simulink model "uz_codegen"  (R2021a)
settings: Solver=FixedStepDiscrete  StartTime=0.0  StopTime=50  RelTol=1e-3  EnableMultiTasking=on
PreLoadFcn:
  | uz_setCodegenPaths
model workspace (MATLAB code in the model file):
  | cmdLim = Simulink.Parameter;
  | cmdLim.Value = 15;
  | cmdLim.Description = 'Limit for controlling the maximum surface command angle.';
  | cmdLim.Min = 0;
  | cmdLim.Max = 90;
  | cmdLim.DocUnits = 'deg';
  | 
  | dispGain = Simulink.Parameter;
  | dispGain.Value = 0.75;
  | dispGain.Description = 'Gain applied to the displacement error.';
  | dispGain.Min = 0;
  | dispGain.Max = [];
  | dispGain.DocUnits = 'deg/sec/deg';
  | 
  | dispLim = Simulink.Parameter;
  | dispLim.Value = 30;
  | dispLim.Description = 'Limit for controlling the maximum commanded angle.';
  | dispLim.Min = 0;
  | dispLim.Max = 180;
  | dispLim.DocUnits = 'deg';
  | 
  | intGain = Simulink.Parameter;
  | intGain.Value = 0.5;
  | intGain.Description = 'Gain applied to the integral error.';
  | intGain.Min = 0;
  | intGain.Max = [];
  | intGain.DocUnits = 'deg/sec/deg/sec';
  | 
  | intLim = Simulink.Parameter;
  | intLim.Value = 5;
  | intLim.Description = 'Limit for controlling the maximum commanded angle.';
  | intLim.Min = 0;
  | intLim.Max = 90;
  | intLim.DocUnits = 'deg';
  | 
  | rateGain = Simulink.Parameter;
  | rateGain.Value = 2;
  | rateGain.Description = 'Gain applied to the rate error.';
  | rateGain.Min = 0;
  | rateGain.Max = [];
  | rateGain.DocUnits = 'deg/deg/sec';
  | 
  | rateLim = Simulink.Parameter;
  | rateLim.Value = 6;
  | rateLim.Description = 'Limit for controlling the maximum commanded angle.';
  | rateLim.Min = 0;
  | rateLim.Max = 180;
  | rateLim.DocUnits = 'deg/sec';
  | 
  | hdgGain = Simulink.Parameter;
  | hdgGain.Value = 0.015;
values from neighbouring files (symbols this model uses):
  I_max = 100    [PMSM_01_Parameter.m]
  Iq_Intersection_Wb = sqrt(I_max^2 - Id_Intersection_Wb^2)    [Plot_MMPA.m]
  Ki_IdController = R/Ld    (= 3749.81250937)    [PMSM_01_Parameter.m]
  Ki_IqController = R/Lq    (= 2500)    [PMSM_01_Parameter.m]
  Ki_SpeedController = Kp_IqController/(Lq*damping_factor^2)    (= 174.532925199)    [PMSM_01_Parameter.m]
  Ki_TorqueController = 1/(4*T_summe_Torque)    (= 714.285714286)    [PMSM_01_Parameter.m]
  Kp_IdController = Ld*2*pi*BW    (= 0.0670239943087)    [PMSM_01_Parameter.m]
  Kp_IqController = Lq*2*pi*BW    (= 0.100530964915)    [PMSM_01_Parameter.m]
  Kp_SpeedController = Kp_IqController/(Lq*damping_factor*K)    (= 2.90111828368)    [PMSM_01_Parameter.m]
  Kp_TorqueController = T1_Torque/(2*T_summe_Torque)    (= 0.373999125427)    [PMSM_01_Parameter.m]
  Ld = 0.6667*Lq    (= 1.06672e-05)    [PMSM_01_Parameter.m]
  List_Iq_Intersection_Speed = zeros(length(List_wEl_Intersection_Speed),1)    [Plot_MMPA.m]
  List_Iq_Torque = zeros(length(List_M_const),1)    [Plot_MMPA.m]
  List_Iq_Torque_Imax = List_Iq_Torque_Imax(List_Iq_Torque_Imax ~= -1)    [Plot_MMPA.m]
  List_M_const = 0:0.5:10    [Plot_MMPA.m]
  List_M_Imax = List_M_const(List_Iq_Torque_Imax ~= -1)    [Plot_MMPA.m]
  List_wEl_Intersection_Speed = linspace(n_cut,n_max,15)    [Plot_MMPA.m]
  Lq = 16e-6    (= 1.6e-05)    [PMSM_01_Parameter.m]
  n_cut = w_b*30/(pi*zp)    [Plot_MMPA.m]
  psi_pm = 0.0030    (= 0.003)    [PMSM_01_Parameter.m]
  R = 0.040    (= 0.04)    [PMSM_01_Parameter.m]
  T_controller = 1/f_CurrentController    (= 0.0001)    [PMSM_01_Parameter.m]
  T_speedController = T_controller    (= 0.0001)    [PMSM_01_Parameter.m]
  U_DC = 46    [PMSM_01_Parameter.m]
  U_maxDQ = U_DC/sqrt(3)    [PMSM_01_Parameter.m]
  zp = 21    [PMSM_01_Parameter.m]
undefined symbols (not defined in the file or in its folder): denum_Gd_speed, denum_Gd_trq, num_Gd_speed, num_Gd_trq
libraries: pid_lib x8, simulink x7, spsabctodq0Lib x2, spsdq0toAlphaBetaZeroLib x2
(part 2 of 2)

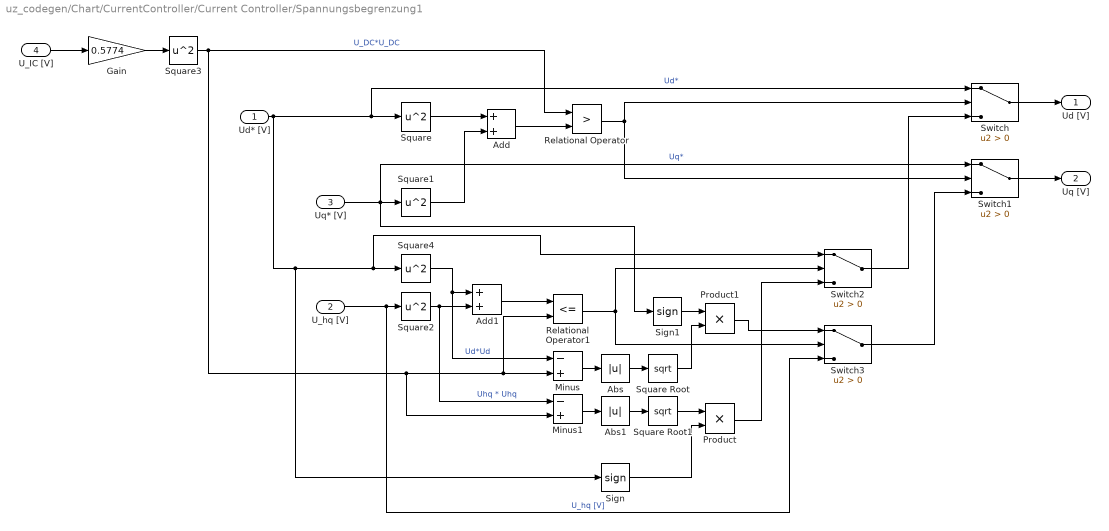
== system uz_codegen/Chart/CurrentController/Current Controller/Spannungsbegrenzung1 ==
  Ud* [V] : Inport
  U_hq [V] : Inport  Port=2
  Uq* [V] : Inport  Port=3
  U_IC [V] : Inport  Port=4
  Abs : Abs
  Abs1 : Abs
  Add : Sum
  Add1 : Sum
  Gain : Gain  Gain=0.5774
  Minus : Sum  Inputs=-+
  Minus1 : Sum  Inputs=-+
  Product : Product
  Product1 : Product
  Relational Operator : RelationalOperator  Operator=>  OutDataTypeStr=boolean  RndMeth=Simplest
  Relational Operator1 : RelationalOperator  Operator=<=  OutDataTypeStr=boolean  RndMeth=Simplest
  Sign : Signum
  Sign1 : Signum
  Square{,1..4} (5 alike) : Math  Operator=square  SaturateOnIntegerOverflow=on
  Square Root : Sqrt  SaturateOnIntegerOverflow=on
  Square Root1 : Sqrt  SaturateOnIntegerOverflow=on
  Switch{,1..3} (4 alike) : Switch  Criteria=u2 > Threshold
  Ud [V] : Outport
  Uq [V] : Outport  Port=2
  wires:
  Ud* [V]/1 -> Sign/1, Switch2/1, Square4/1, Switch/1, Square/1  "Ud*"
  Uq* [V]/1 -> Switch1/1, Sign1/1, Square1/1  "Uq*"
  U_hq [V]/1 -> Switch3/3, Square2/1  "U_hq [V]"
  U_IC [V]/1 -> Gain/1
  Square1/1 -> Add/2
  Square/1 -> Add/1
  Square3/1 -> Minus1/2, Minus/2, Relational Operator1/2, Relational Operator/1  "U_DC*U_DC"
  Add/1 -> Relational Operator/2
  Switch/1 -> Ud [V]/1
  Relational Operator/1 -> Switch1/2, Switch/2
  Switch1/1 -> Uq [V]/1
  Square2/1 -> Minus1/1, Add1/2  "Uhq * Uhq"
  Square4/1 -> Minus/1, Add1/1  "Ud*Ud"
  Add1/1 -> Relational Operator1/1
  Relational Operator1/1 -> Switch2/2, Switch3/2
  Switch2/1 -> Switch/3
  Switch3/1 -> Switch1/3
  Minus/1 -> Abs/1
  Square Root/1 -> Product1/2
  Minus1/1 -> Abs1/1
  Square Root1/1 -> Product/1
  Abs1/1 -> Square Root1/1
  Abs/1 -> Square Root/1
  Gain/1 -> Square3/1
  Sign/1 -> Product/2
  Product/1 -> Switch2/3
  Sign1/1 -> Product1/1
  Product1/1 -> Switch3/1

== system uz_codegen/Chart/SpeedController/speed controller/MMPA_Controller ==
  flg_speedControl : Inport
  n_soll : Inport  Port=2
  n_ist : Inport  Port=3
  id_ref : Inport  Port=4
  iq_ref : Inport  Port=5
  Discrete Transfer Fcn : DiscreteTransferFcn  Numerator=num_Gd_trq  Denominator=denum_Gd_trq
  PID Controller : pid_lib/PID Controller  Controller=PI  Form=Ideal  TimeDomain=Discrete-time  UseExternalTs=off  SampleTime=-1  IntegratorMethod=Forward Euler  FilterMethod=Forward Euler  ControllerParametersSource=internal  P=Kp_TorqueController  I=Ki_TorqueController  D=0  UseFilter=on  N=100  TunerSelectOption=Transfer Function Based (PID Tuner App)  InitialConditionSource=internal  InitialConditionForIntegrator=0  InitialConditionForFilter=0  DifferentiatorICPrevScaledInput=0  ExternalReset=none  TrackingMode=off  Kt=1  LimitOutput=on  SatLimitsSource=internal  UpperSaturationLimit=8  LowerSaturationLimit=-8  LinearizeAsGain=on  AntiWindupMode=clamping  Kb=1  POutMin=[]  POutMax=[]  IOutMin=[]  IOutMax=[]  DOutMin=[]  DOutMax=[]  NOutMin=[]  NOutMax=[]  SumOutMin=[]  SumOutMax=[]  SaturationOutMin=[]  SaturationOutMax=[]  PParamMin=[]  PParamMax=[]  IParamMin=[]  IParamMax=[]  DParamMin=[]  DParamMax=[]  NParamMin=[]  NParamMax=[]  KbParamMin=[]  KbParamMax=[]  KtParamMin=[]  KtParamMax=[]  KbOutMin=[]  KbOutMax=[]  KtOutMin=[]  KtOutMax=[]  IntegratorOutMin=[]  IntegratorOutMax=[]  FilterOutMin=[]  FilterOutMax=[]  SumI1OutMin=[]  SumI1OutMax=[]  SumI2OutMin=[]  SumI2OutMax=[]  SumI3OutMin=[]  SumI3OutMax=[]  SumI4OutMin=[]  SumI4OutMax=[]  SumDOutMin=[]  SumDOutMax=[]  DifferentiatorOutMin=[]  DifferentiatorOutMax=[]  FilterDiffOutCoefMin=[]  FilterDiffOutCoefMax=[]  ReciprocalOutMin=[]  ReciprocalOutMax=[]  SumDenOutMin=[]  SumDenOutMax=[]  SumNumOutMin=[]  SumNumOutMax=[]  DivideOutMin=[]  DivideOutMax=[]  UdiffTsProdOutMin=[]  UdiffTsProdOutMax=[]  NTsProdOutMin=[]  NTsProdOutMax=[]  UintegralTsProdOutMin=[]  UintegralTsProdOutMax=[]  UngainTsProdOutMin=[]  UngainTsProdOutMax=[]  IntegratorContinuousStateAttributes=''  IntegratorStateMustResolveToSignalObject=off  IntegratorRTWStateStorageClass=Auto  FilterContinuousStateAttributes=''  FilterStateMustResolveToSignalObject=off  FilterRTWStateStorageClass=Auto  ParallelPVariant=Passthrough  IdealPVariant=InternalParameters  IVariant=InternalParameters  DVariant=Disabled  IntegratorVariant=Discrete  SatVariant=Enabled  AWVariant=DiscClampingIdeal  PCopyVariant=InternalParamsIdeal  TRVariant=Disabled  FdbkBlocksVariant=Forward  IdealPFdbkVariant=Disabled  SatFdbkVariant=Disabled  DerivativeFilterVariant=Disabled  NVariant=Disabled  NCopyVariant=Disabled_SignalSpec  FilterICVariant=Disabled  IntegratorICVariant=InternalICs  ExternalResetVariant=Disabled  TRSumVariant=Passthrough  SumFdbkVariant=Disabled  SumVariant=Sum_PI  TsampFilterVariant=InternalTs  TsampNgainVariant=Passthrough  TsampIntegralVariant=Passthrough  ExternalSaturationOutDataTypeStr=Inherit: Same as second input
  Scope : Scope  NumInputPorts=2
  Scope1 : Scope
  Subsystem : Subsystem
  Sum : Sum  Inputs=|+-
  Switch : Switch  Criteria=u2 > Threshold
  Switch1 : Switch  Criteria=u2 > Threshold
  id_soll : Outport
  Iq_soll : Outport  Port=2
  wires:
  Subsystem/1(Iq) -> Scope/1, Switch1/1
  PID Controller/1 -> Scope1/1, Subsystem/1(M_soll)  "M_soll"
  n_soll/1 -> Discrete Transfer Fcn/1
  flg_speedControl/1 -> Switch/2, Switch1/2
  n_ist/1 -> Sum/2, Subsystem/2(n_ist)
  iq_ref/1 -> Switch1/3
  id_ref/1 -> Switch/3
  Sum/1 -> PID Controller/1
  Subsystem/2(Id) -> Scope/2, Switch/1
  Discrete Transfer Fcn/1 -> Sum/1
  Switch1/1 -> Iq_soll/1
  Switch/1 -> id_soll/1

== system uz_codegen/Chart/SpeedController/speed controller/Subsystem ==
  flg_fieldWeakening : Inport
  id_ref : Inport  Port=2
  n_soll : Inport  Port=3
  flg_speedControl : Inport  Port=4
  n_ist : Inport  Port=5
  iq_ref : Inport  Port=6
  Constant : Constant  Value=0
  PID Controller : pid_lib/PID Controller  Controller=PI  Form=Ideal  TimeDomain=Discrete-time  UseExternalTs=off  SampleTime=-1  IntegratorMethod=Forward Euler  FilterMethod=Forward Euler  ControllerParametersSource=internal  P=Kp_SpeedController  I=Ki_SpeedController  D=0  UseFilter=on  N=100  TunerSelectOption=Transfer Function Based (PID Tuner App)  InitialConditionSource=internal  InitialConditionForIntegrator=0  InitialConditionForFilter=0  DifferentiatorICPrevScaledInput=0  ExternalReset=none  TrackingMode=off  Kt=1  LimitOutput=on  SatLimitsSource=internal  UpperSaturationLimit=I_max  LowerSaturationLimit=-I_max  LinearizeAsGain=on  AntiWindupMode=clamping  Kb=1  POutMin=[]  POutMax=[]  IOutMin=[]  IOutMax=[]  DOutMin=[]  DOutMax=[]  NOutMin=[]  NOutMax=[]  SumOutMin=[]  SumOutMax=[]  SaturationOutMin=[]  SaturationOutMax=[]  PParamMin=[]  PParamMax=[]  IParamMin=[]  IParamMax=[]  DParamMin=[]  DParamMax=[]  NParamMin=[]  NParamMax=[]  KbParamMin=[]  KbParamMax=[]  KtParamMin=[]  KtParamMax=[]  KbOutMin=[]  KbOutMax=[]  KtOutMin=[]  KtOutMax=[]  IntegratorOutMin=[]  IntegratorOutMax=[]  FilterOutMin=[]  FilterOutMax=[]  SumI1OutMin=[]  SumI1OutMax=[]  SumI2OutMin=[]  SumI2OutMax=[]  SumI3OutMin=[]  SumI3OutMax=[]  SumI4OutMin=[]  SumI4OutMax=[]  SumDOutMin=[]  SumDOutMax=[]  DifferentiatorOutMin=[]  DifferentiatorOutMax=[]  FilterDiffOutCoefMin=[]  FilterDiffOutCoefMax=[]  ReciprocalOutMin=[]  ReciprocalOutMax=[]  SumDenOutMin=[]  SumDenOutMax=[]  SumNumOutMin=[]  SumNumOutMax=[]  DivideOutMin=[]  DivideOutMax=[]  UdiffTsProdOutMin=[]  UdiffTsProdOutMax=[]  NTsProdOutMin=[]  NTsProdOutMax=[]  UintegralTsProdOutMin=[]  UintegralTsProdOutMax=[]  UngainTsProdOutMin=[]  UngainTsProdOutMax=[]  IntegratorContinuousStateAttributes=''  IntegratorStateMustResolveToSignalObject=off  IntegratorRTWStateStorageClass=Auto  FilterContinuousStateAttributes=''  FilterStateMustResolveToSignalObject=off  FilterRTWStateStorageClass=Auto  ParallelPVariant=Passthrough  IdealPVariant=InternalParameters  IVariant=InternalParameters  DVariant=Disabled  IntegratorVariant=Discrete  SatVariant=Enabled  AWVariant=DiscClampingIdeal  PCopyVariant=InternalParamsIdeal  TRVariant=Disabled  FdbkBlocksVariant=Forward  IdealPFdbkVariant=Disabled  SatFdbkVariant=Disabled  DerivativeFilterVariant=Disabled  NVariant=Disabled  NCopyVariant=Disabled_SignalSpec  FilterICVariant=Disabled  IntegratorICVariant=InternalICs  ExternalResetVariant=Disabled  TRSumVariant=Passthrough  SumFdbkVariant=Disabled  SumVariant=Sum_PI  TsampFilterVariant=InternalTs  TsampNgainVariant=Passthrough  TsampIntegralVariant=Passthrough  ExternalSaturationOutDataTypeStr=Inherit: Same as second input
  Sum : Sum  Inputs=|+-
  Switch : Switch  Criteria=u2 > Threshold
  Switch1 : Switch  Criteria=u2 > Threshold
  id_soll : Outport
  iq_soll : Outport  Port=2
  wires:
  iq_ref/1 -> Switch1/3
  n_ist/1 -> Sum/2
  id_ref/1 -> Switch/3
  flg_fieldWeakening/1 -> Switch/2
  PID Controller/1 -> Switch1/1
  Sum/1 -> PID Controller/1
  flg_speedControl/1 -> Switch1/2
  n_soll/1 -> Sum/1
  Switch/1 -> id_soll/1
  Switch1/1 -> iq_soll/1
  Constant/1 -> Switch/1

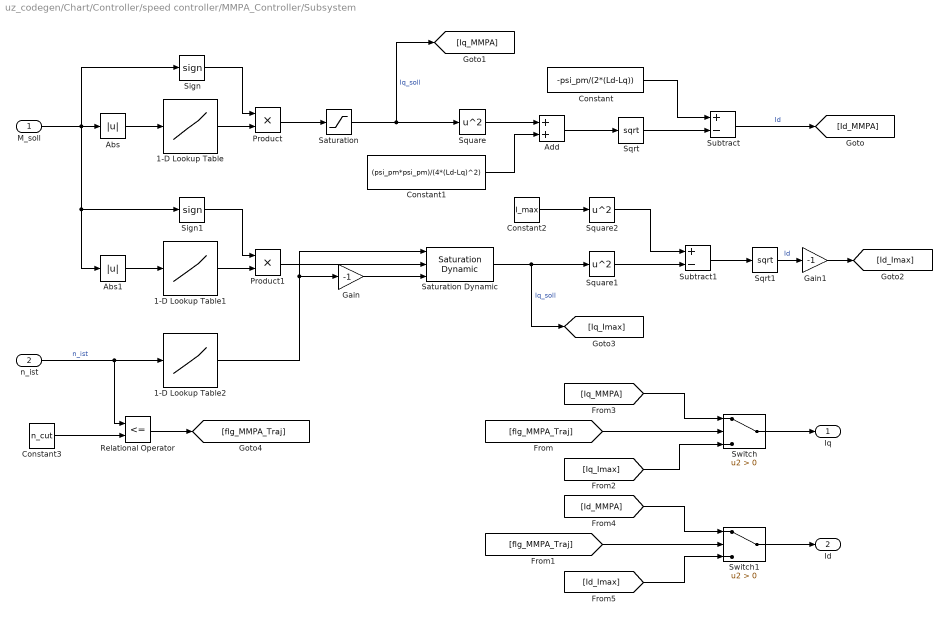
== system uz_codegen/Chart/Controller/speed controller/MMPA_Controller/Subsystem ==
  M_soll : Inport
  n_ist : Inport  Port=2
  1-D Lookup Table : Lookup_n-D  NumberOfTableDimensions=1  BreakpointsForDimension1=List_M_const  Table=List_Iq_Torque  InternalRulePriority=Speed  RndMeth=Simplest  InputSameDT=on
  1-D Lookup Table1 : Lookup_n-D  NumberOfTableDimensions=1  BreakpointsForDimension1=List_M_Imax  Table=List_Iq_Torque_Imax  InternalRulePriority=Speed  RndMeth=Simplest  InputSameDT=on
  1-D Lookup Table2 : Lookup_n-D  NumberOfTableDimensions=1  BreakpointsForDimension1=List_wEl_Intersection_Speed  Table=List_Iq_Intersection_Speed  InternalRulePriority=Speed  RndMeth=Simplest  InputSameDT=on
  Abs : Abs
  Abs1 : Abs
  Add : Sum
  Constant : Constant  Value=-psi_pm/(2*(Ld-Lq))
  Constant1 : Constant  Value=(psi_pm*psi_pm)/(4*(Ld-Lq)^2)
  Constant2 : Constant  Value=I_max
  Constant3 : Constant  Value=n_cut
  Gain : Gain  Gain=-1
  Gain1 : Gain  Gain=-1
  Product : Product
  Product1 : Product
  Relational Operator : RelationalOperator  Operator=<=  OutDataTypeStr=boolean  RndMeth=Simplest
  Saturation : Saturate  UpperLimit=Iq_Intersection_Wb  LowerLimit=-Iq_Intersection_Wb
  Saturation Dynamic : simulink/Discontinuities/Saturation Dynamic  OutMin=[]  OutMax=[]  OutDataTypeStr=Inherit: Same as second input  OutDataType=fixdt(1, 16)  OutScaling=2^-10  DoSatur=off
  Sign : Signum
  Sign1 : Signum
  Sqrt : Sqrt  SaturateOnIntegerOverflow=on
  Sqrt1 : Sqrt  SaturateOnIntegerOverflow=on
  Square : Math  Operator=square  SaturateOnIntegerOverflow=on
  Square1 : Math  Operator=square  SaturateOnIntegerOverflow=on
  Square2 : Math  Operator=square  SaturateOnIntegerOverflow=on
  Subtract : Sum  Inputs=+-
  Subtract1 : Sum  Inputs=+-
  Switch : Switch  Criteria=u2 > Threshold
  Switch1 : Switch  Criteria=u2 > Threshold
  Iq : Outport
  Id : Outport  Port=2
  wires:
  1-D Lookup Table/1 -> Product/2
  Abs/1 -> 1-D Lookup Table/1
  Product/1 -> Saturation/1
  Sign/1 -> Product/1
  Saturation/1 -> [Iq_MMPA], Square/1  "Iq_soll"
  Square/1 -> Add/1
  Constant1/1 -> Add/2
  Add/1 -> Sqrt/1
  Sqrt/1 -> Subtract/2
  Constant/1 -> Subtract/1
  Subtract/1 -> [Id_MMPA]  "Id"
  Abs1/1 -> 1-D Lookup Table1/1
  Sign1/1 -> Product1/1
  Product1/1 -> Saturation Dynamic/2
  M_soll/1 -> Abs/1, Sign1/1, Abs1/1, Sign/1
  1-D Lookup Table1/1 -> Product1/2
  n_ist/1 -> Relational Operator/1, 1-D Lookup Table2/1  "n_ist"
  1-D Lookup Table2/1 -> Gain/1, Saturation Dynamic/1
  Gain/1 -> Saturation Dynamic/3
  Saturation Dynamic/1 -> [Iq_Imax], Square1/1  "Iq_soll"
  Constant2/1 -> Square2/1
  Square1/1 -> Subtract1/2
  Square2/1 -> Subtract1/1
  Subtract1/1 -> Sqrt1/1
  Sqrt1/1 -> Gain1/1  "Id"
  Constant3/1 -> Relational Operator/2
  Relational Operator/1 -> [flg_MMPA_Traj]
  [flg_MMPA_Traj] -> Switch/2
  [flg_MMPA_Traj] -> Switch1/2
  [Iq_Imax] -> Switch/3
  [Iq_MMPA] -> Switch/1
  [Id_MMPA] -> Switch1/1
  [Id_Imax] -> Switch1/3
  Switch1/1 -> Id/1
  Switch/1 -> Iq/1
  Gain1/1 -> [Id_Imax]

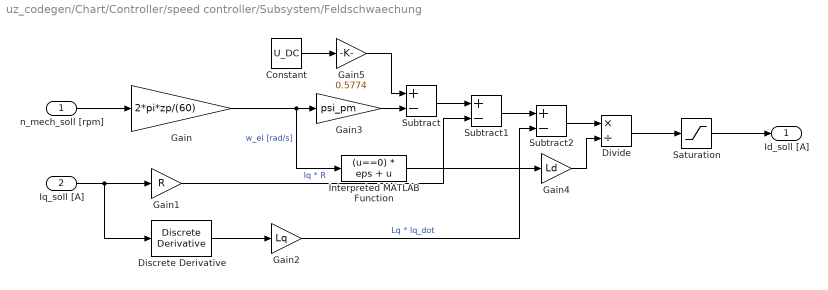
== system uz_codegen/Chart/Controller/speed controller/Subsystem/Feldschwaechung ==
  n_mech_soll [rpm] : Inport
  Iq_soll [A] : Inport  Port=2
  Constant : Constant  Value=U_DC
  Discrete Derivative : simulink/Discrete/Discrete Derivative  gainval=1.0  ICPrevScaledInput=0.0  OutMin=[]  OutMax=[]  OutDataType=fixdt(1, 16)  OutScaling=2^-10  DoSatur=off
  Divide : Product  Inputs=*/
  Gain : Gain  Gain=2*pi*zp/(60)
  Gain1 : Gain  Gain=R
  Gain2 : Gain  Gain=Lq
  Gain3 : Gain  Gain=psi_pm
  Gain4 : Gain  Gain=Ld
  Gain5 : Gain  Gain=0.5774
  Interpreted MATLAB Function : MATLABFcn  MATLABFcn=(u==0) * eps + u
  Saturation : Saturate  UpperLimit=0  LowerLimit=-I_max
  Subtract : Sum  Inputs=+-
  Subtract1 : Sum  Inputs=+-
  Subtract2 : Sum  Inputs=+-
  Id_soll [A] : Outport
  wires:
  n_mech_soll [rpm]/1 -> Gain/1
  Gain/1 -> Interpreted MATLAB Function/1, Gain3/1  "w_el [rad/s]"
  Gain1/1 -> Subtract1/2  "Iq * R"
  Iq_soll [A]/1 -> Discrete Derivative/1, Gain1/1
  Discrete Derivative/1 -> Gain2/1
  Gain2/1 -> Subtract2/2  "Lq * Iq_dot"
  Constant/1 -> Gain5/1
  Subtract/1 -> Subtract1/1
  Subtract1/1 -> Subtract2/1
  Subtract2/1 -> Divide/1
  Gain3/1 -> Subtract/2
  Gain4/1 -> Divide/2
  Divide/1 -> Saturation/1
  Saturation/1 -> Id_soll [A]/1
  Interpreted MATLAB Function/1 -> Gain4/1
  Gain5/1 -> Subtract/1

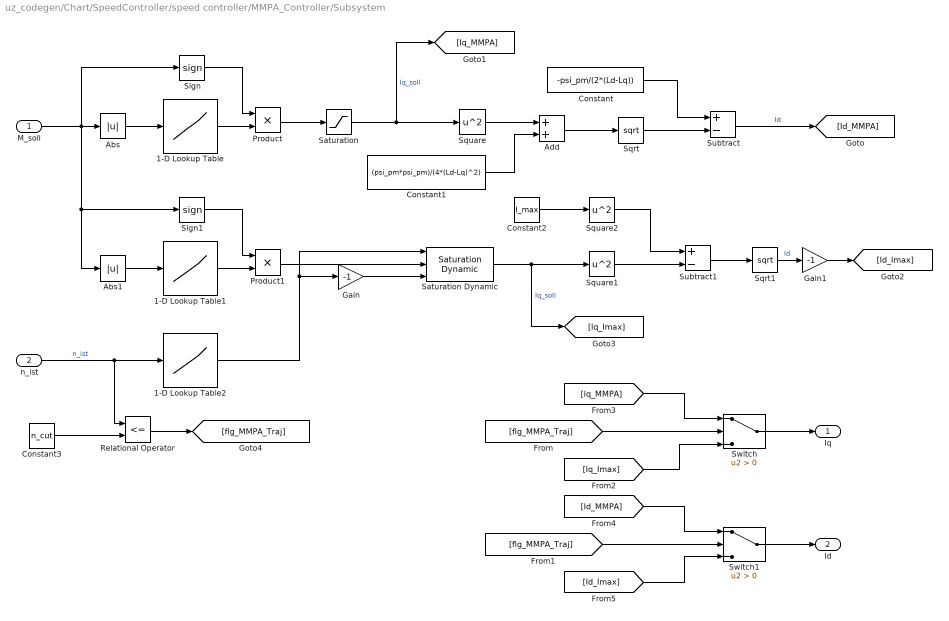
== system uz_codegen/Chart/SpeedController/speed controller/MMPA_Controller/Subsystem ==
  M_soll : Inport
  n_ist : Inport  Port=2
  1-D Lookup Table : Lookup_n-D  NumberOfTableDimensions=1  BreakpointsForDimension1=List_M_const  Table=List_Iq_Torque  InternalRulePriority=Speed  RndMeth=Simplest  InputSameDT=on
  1-D Lookup Table1 : Lookup_n-D  NumberOfTableDimensions=1  BreakpointsForDimension1=List_M_Imax  Table=List_Iq_Torque_Imax  InternalRulePriority=Speed  RndMeth=Simplest  InputSameDT=on
  1-D Lookup Table2 : Lookup_n-D  NumberOfTableDimensions=1  BreakpointsForDimension1=List_wEl_Intersection_Speed  Table=List_Iq_Intersection_Speed  InternalRulePriority=Speed  RndMeth=Simplest  InputSameDT=on
  Abs : Abs
  Abs1 : Abs
  Add : Sum
  Constant : Constant  Value=-psi_pm/(2*(Ld-Lq))
  Constant1 : Constant  Value=(psi_pm*psi_pm)/(4*(Ld-Lq)^2)
  Constant2 : Constant  Value=I_max
  Constant3 : Constant  Value=n_cut
  Gain : Gain  Gain=-1
  Gain1 : Gain  Gain=-1
  Product : Product
  Product1 : Product
  Relational Operator : RelationalOperator  Operator=<=  OutDataTypeStr=boolean  RndMeth=Simplest
  Saturation : Saturate  UpperLimit=Iq_Intersection_Wb  LowerLimit=-Iq_Intersection_Wb
  Saturation Dynamic : simulink/Discontinuities/Saturation Dynamic  OutMin=[]  OutMax=[]  OutDataTypeStr=Inherit: Same as second input  OutDataType=fixdt(1, 16)  OutScaling=2^-10  DoSatur=off
  Sign : Signum
  Sign1 : Signum
  Sqrt : Sqrt  SaturateOnIntegerOverflow=on
  Sqrt1 : Sqrt  SaturateOnIntegerOverflow=on
  Square : Math  Operator=square  SaturateOnIntegerOverflow=on
  Square1 : Math  Operator=square  SaturateOnIntegerOverflow=on
  Square2 : Math  Operator=square  SaturateOnIntegerOverflow=on
  Subtract : Sum  Inputs=+-
  Subtract1 : Sum  Inputs=+-
  Switch : Switch  Criteria=u2 > Threshold
  Switch1 : Switch  Criteria=u2 > Threshold
  Iq : Outport
  Id : Outport  Port=2
  wires:
  1-D Lookup Table/1 -> Product/2
  Abs/1 -> 1-D Lookup Table/1
  Product/1 -> Saturation/1
  Sign/1 -> Product/1
  Saturation/1 -> [Iq_MMPA], Square/1  "Iq_soll"
  Square/1 -> Add/1
  Constant1/1 -> Add/2
  Add/1 -> Sqrt/1
  Sqrt/1 -> Subtract/2
  Constant/1 -> Subtract/1
  Subtract/1 -> [Id_MMPA]  "Id"
  Abs1/1 -> 1-D Lookup Table1/1
  Sign1/1 -> Product1/1
  Product1/1 -> Saturation Dynamic/2
  M_soll/1 -> Abs/1, Sign1/1, Abs1/1, Sign/1
  1-D Lookup Table1/1 -> Product1/2
  n_ist/1 -> Relational Operator/1, 1-D Lookup Table2/1  "n_ist"
  1-D Lookup Table2/1 -> Gain/1, Saturation Dynamic/1
  Gain/1 -> Saturation Dynamic/3
  Saturation Dynamic/1 -> [Iq_Imax], Square1/1  "Iq_soll"
  Constant2/1 -> Square2/1
  Square1/1 -> Subtract1/2
  Square2/1 -> Subtract1/1
  Subtract1/1 -> Sqrt1/1
  Sqrt1/1 -> Gain1/1  "Id"
  Constant3/1 -> Relational Operator/2
  Relational Operator/1 -> [flg_MMPA_Traj]
  [flg_MMPA_Traj] -> Switch/2
  [flg_MMPA_Traj] -> Switch1/2
  [Iq_Imax] -> Switch/3
  [Iq_MMPA] -> Switch/1
  [Id_MMPA] -> Switch1/1
  [Id_Imax] -> Switch1/3
  Switch1/1 -> Id/1
  Switch/1 -> Iq/1
  Gain1/1 -> [Id_Imax]

== matlab function uz_codegen/Chart/Controller/SpaceVectorModulation/SpaceVectorModulation ==
  data: u_alpha input; u_a output; u_beta input; U_ZK input; u_b output; u_c output; sector output
function [u_a, u_b, u_c, sector] = fcn(u_alpha, u_beta, U_ZK)

a_U_on=0;
a_V_on=0;
a_W_on=0;

 %%__%%__%%__%%__%%__%%__%%__%%__%%__%%__%%__%%__%%__%%__%%__%%__%%__%%__%%_
    %%Trägerbasierte Raumzeigermodulation%%
    %%Eingänge:
    %U_ZK       -- Zwischenkreisspannung
    %u_alpha    -- alphakomponente des Sollspannungsraumzeigers
    %u_beta     -- betakomponente des Sollspannungsraumzeigers
    %CMP_Period_max_val  -- maximalwert des Dreiecks/Sägezahnzählers zum Gewichten der Aussteuergrade
    %%Ausgänge:
    %CMP_U        -- Vergleichswert U
    %CMP_V        -- Vergleichswert V
    %CMP_W        -- Vergleichswert W
    %sector       -- Ausgabe des Sektors des Spannungszeigers
    
    
    %Berechnung von a, b, c nach Quang Dittrich S24
    
    a = abs(u_alpha) + 0.5774*abs(u_beta);
    b = abs(u_alpha) - 0.5774*abs(u_beta);
    c = 1.1547*abs(u_beta);
    
    U_max = 0.6667 * U_ZK; %Maximum Voltage U_ZL/sqrt(3)
    
    
    %Sektor und Quadranten nach Quang Dittrich S32
    if(u_beta < 0)
        if (u_alpha <0)
            quadrant=3;
            if(b < 0)
                sector = 5;
            else
                sector = 4;
            end
        else
            quadrant=4;
            if(b < 0)
                sector = 5;
            else
                sector = 6;
            end
        end
        
    else
        if (u_alpha <0)
            quadrant=2;
            if(b < 0)
                sector = 2;
            else
                sector = 3;
            end
        else
            quadrant=1;
            if(b < 0)
                sector = 2;
            else
                sector = 1;
            end
        end
    end
    
    sector = sector;
    
    %%Modulationsfunktionen für Phasen U,V,W
    %%Erzeugung der Aussteuergrade für die Halbbrücken
    %%--> Erzeugung einer "regulary Sampled SVM" erfolgt anschließend durch Abtastung
    %%mit Dreieckszählern in Hardware.
    
    if (sector == 1)
        
        %Quang S.24 and normed to 2/3 U_DC
        u1 = b/(U_max);
        u2 = c/(U_max);
        
        %Quang S.34
        a_U_on = 0.5 + u1*0.5 + u2*0.5;
        a_V_on = 0.5 - u1*0.5 + u2*0.5;
        a_W_on = 0.5 - u1*0.5 - u2*0.5;
    end
    
    
    if ((sector == 2) && (quadrant == 1))
        
        u1 = a/(U_max);
        u2 = (-abs(u_alpha) + 0.5774*abs(u_beta))/(U_max);
        
        a_U_on = 0.5 + u1*0.5 - u2*0.5;
        a_V_on = 0.5 + u1*0.5 + u2*0.5;
        a_W_on = 0.5 - u1*0.5 - u2*0.5;
    end
    
    
    if ((sector == 2) && (quadrant == 2))
        
        u1 = (-abs(u_alpha) + 0.5774*abs(u_beta))/(U_max);
        u2 = a/(U_max);
        
        a_U_on = 0.5 + u1*0.5 - u2*0.5;
        a_V_on = 0.5 + u1*0.5 + u2*0.5;
        a_W_on = 0.5 - u1*0.5 - u2*0.5;
    end
    
    
    if (sector == 3)
        
        u1 = c/(U_max);
        u2 = b/(U_max);
        
        a_U_on=  0.5 - u1*0.5 - u2*0.5;
        a_V_on = 0.5 + u1*0.5 + u2*0.5;
        a_W_on = 0.5 - u1*0.5 + u2*0.5;
    end
    
    if (sector == 4)
        
        u1 = b/(U_max);
        u2 = c/(U_max);
        
        a_U_on = 0.5 - u1*0.5 - u2*0.5;
        a_V_on = 0.5 + u1*0.5 - u2*0.5;
        a_W_on = 0.5 + u1*0.5 + u2*0.5;
    end
    
    
    if ((sector == 5) && (quadrant == 3))
        
        u1 = a/(U_max);
        u2 = (-abs(u_alpha) + 0.5774*abs(u_beta))/(U_max);
        
        a_U_on = 0.5 - u1*0.5 + u2*0.5;
        a_V_on = 0.5 - u1*0.5 - u2*0.5;
        a_W_on = 0.5 + u1*0.5 + u2*0.5;
    end
    
    
    if ((sector == 5) && (quadrant == 4))
        
        u1 =(-abs(u_alpha) + 0.5774*abs(u_beta))/(U_max);
        u2 =  a/(U_max);
        
        a_U_on = 0.5 - u1*0.5 + u2*0.5;
        a_V_on = 0.5 - u1*0.5 - u2*0.5;
        a_W_on = 0.5 + u1*0.5 + u2*0.5;
    end
    
    
    if (sector == 6)
        
        u1 = c/(U_max);
        u2 = b/(U_max);
        
        a_U_on = 0.5 + u1*0.5 + u2*0.5;
        a_V_on = 0.5 - u1*0.5 - u2*0.5;
        a_W_on = 0.5 + u1*0.5 - u2*0.5;
    end
    
    if a_U_on > 1.0
        a_U_on = 1.0;
    end
    if a_V_on > 1.0
        a_V_on = 1.0;
    end
    if a_W_on > 1.0
        a_W_on = 1.0;
    end     
        
    u_a = a_U_on;
    u_b = a_V_on;
    u_c = a_W_on;

== stateflow chart uz_codegen/Chart ==
  state Start
    entry:
    activeState = 1;
    Ua_DutyCycle = 0;
    Ub_DutyCycle = 0;
    Uc_DutyCycle = 0;
  state InProcess
    entry:
    activeState = 2;
    id_soll = 0;
    iq_soll = 0;
    rat_freq = T_speedController/T_controller;
    %during:
    %[Ua_DutyCycle, Ub_DutyCycle, Uc_DutyCycle, iq_ist, id_ist, ud, uq] = Controller(ia, ib, ic, w_el, flg_PreCntr, theta_el, U_IC, iq_ref, id_ref, n_soll, n_ist, flg_fieldWeakening, flg_SpeedControl, flgLimitUdUq,flg_UseMMPA)
    %on every(T_speedController,sec): [id_soll,iq_soll] = SpeedController(id_ref,iq_ref,n_soll,n_ist,flg_fieldWeakening,flg_UseMMPA,flg_SpeedControl);
    %on every(T_controller,sec): [Ua_DutyCycle, Ub_DutyCycle, Uc_DutyCycle, iq_ist, id_ist, ud, uq] = CurrentController(ia, ib, ic, w_el, flg_PreCntr, theta_el, U_IC,id_soll,iq_soll,flgLimitUdUq);
    state CurrentControl
      entry:
      [Ua_DutyCycle, Ub_DutyCycle, Uc_DutyCycle, iq_ist, id_ist, ud, uq] = CurrentController(ia, ib, ic, w_el, flg_PreCntr, theta_el, U_IC,id_soll,iq_soll,flgLimitUdUq)
      cnt_CurrentCtrl = cnt_CurrentCtrl +1;
      during:
      [Ua_DutyCycle, Ub_DutyCycle, Uc_DutyCycle, iq_ist, id_ist, ud, uq] = CurrentController(ia, ib, ic, w_el, flg_PreCntr, theta_el, U_IC,id_soll,iq_soll,flgLimitUdUq)
      cnt_CurrentCtrl = cnt_CurrentCtrl +1;
    state SpeedControl
      entry:
      [id_soll,iq_soll] = SpeedController(id_ref,iq_ref,n_soll,n_ist,flg_fieldWeakening,flg_UseMMPA,flg_SpeedControl)
      [Ua_DutyCycle, Ub_DutyCycle, Uc_DutyCycle, iq_ist, id_ist, ud, uq] = CurrentController(ia, ib, ic, w_el, flg_PreCntr, theta_el, U_IC,id_soll,iq_soll,flgLimitUdUq)
      cnt_CurrentCtrl = 1
      during:
      [id_soll,iq_soll] = SpeedController(id_ref,iq_ref,n_soll,n_ist,flg_fieldWeakening,flg_UseMMPA,flg_SpeedControl)
      [Ua_DutyCycle, Ub_DutyCycle, Uc_DutyCycle, iq_ist, id_ist, ud, uq] = CurrentController(ia, ib, ic, w_el, flg_PreCntr, theta_el, U_IC,id_soll,iq_soll,flgLimitUdUq)
    (default) -> SpeedControl
    CurrentControl -> SpeedControl : [cnt_CurrentCtrl >= rat_freq]
    SpeedControl -> CurrentControl : [rat_freq > 1]
  state [ua,ub,uc,Iq_ist,Id_ist,ud_soll,uq_soll] = CurrentController(ia,ib,ic,w_el,flg_PreCtrl,theta_el,U_IC,id_ref,iq_ref,flg_LimitUdUq) [function]
  state [id_soll, iq_soll] = SpeedController(id_ref,iq_ref,n_soll,n_ist,flg_fieldWeakening,flg_UseMMPA,flg_SpeedControl) [function]
  state [ua,ub,uc,iq_ist,id_ist,ud_soll,uq_soll] = Controller(ia,ib,ic,w_el,flg_Precontroller,theta_el,U_IC,iq_ref,id_ref,n_soll,n_ist,flg_fieldWeakening,flg_SpeedControl,flgLimitUdUq,flg_UseMMPA) [function] [commented out]
  (default) -> Start
  InProcess -> Start : [RESET==1]
  Start -> InProcess : [START==1 & RESET==0]
  data: ia function_input double size=1; ib function_input double size=1; ic function_input double size=1; w_el function_input double size=1; flg_PreCtrl function_input double size=1; theta_el function_input double size=1; ua function_output; ub function_output; uc function_output; Iq_ist function_output; Id_ist function_output; ud_soll function_output; uq_soll function_output; U_IC function_input double size=1; id_ref function_input double size=1; iq_ref function_input double size=1; flg_LimitUdUq function_input double size=1; id_ref function_input double size=1; iq_ref function_input double size=1; n_soll function_input double size=1; n_ist function_input double size=1; flg_fieldWeakening function_input double size=1; flg_UseMMPA function_input double size=1; flg_SpeedControl function_input double size=1; id_soll function_output; iq_soll function_output; ia function_input double size=1; ib function_input double size=1; ic function_input double size=1; ua function_output double size=1; ub function_output double size=1; uc function_output double size=1; iq_ist function_output double size=1; id_ist function_output double size=1; w_el function_input double size=1; flg_Precontroller function_input double size=1; theta_el function_input double size=1; U_IC function_input double size=1; iq_ref function_input double size=1; id_ref function_input double size=1; n_soll function_input double size=1; n_ist function_input double size=1; flg_fieldWeakening function_input double size=1; flg_SpeedControl function_input double size=1; ud_soll function_output double size=1; uq_soll function_output double size=1; flgLimitUdUq function_input double size=1; flg_UseMMPA function_input double size=1; flg_PreCntr input; flg_fieldWeakening input; flg_SpeedControl input; ic input; ib input; w_el input; ia input; theta_el input; iq_ref input; n_ist input; id_ref input; n_soll input; Ua_DutyCycle output; activeState output; Uc_DutyCycle output; Ub_DutyCycle output; iq_ist output; id_ist output; U_IC input; RESET input; START input; uq output; ud output; flgLimitUdUq input; flg_UseMMPA input; T_speedController input; T_controller input; id_soll local; iq_soll local; rat_freq local; cnt_CurrentCtrl local

== matlab function uz_codegen/Chart/CurrentController/SpaceVectorModulation/SpaceVectorModulation ==
  data: u_alpha input; u_a output; u_beta input; U_ZK input; u_b output; u_c output; sector output
function [u_a, u_b, u_c, sector] = fcn(u_alpha, u_beta, U_ZK)

a_U_on=0;
a_V_on=0;
a_W_on=0;

 %%__%%__%%__%%__%%__%%__%%__%%__%%__%%__%%__%%__%%__%%__%%__%%__%%__%%__%%_
    %%Trägerbasierte Raumzeigermodulation%%
    %%Eingänge:
    %U_ZK       -- Zwischenkreisspannung
    %u_alpha    -- alphakomponente des Sollspannungsraumzeigers
    %u_beta     -- betakomponente des Sollspannungsraumzeigers
    %CMP_Period_max_val  -- maximalwert des Dreiecks/Sägezahnzählers zum Gewichten der Aussteuergrade
    %%Ausgänge:
    %CMP_U        -- Vergleichswert U
    %CMP_V        -- Vergleichswert V
    %CMP_W        -- Vergleichswert W
    %sector       -- Ausgabe des Sektors des Spannungszeigers
    
    
    %Berechnung von a, b, c nach Quang Dittrich S24
    
    a = abs(u_alpha) + 0.5774*abs(u_beta);
    b = abs(u_alpha) - 0.5774*abs(u_beta);
    c = 1.1547*abs(u_beta);
    
    U_max = 0.6667 * U_ZK; %Maximum Voltage U_ZL/sqrt(3)
    
    
    %Sektor und Quadranten nach Quang Dittrich S32
    if(u_beta < 0)
        if (u_alpha <0)
            quadrant=3;
            if(b < 0)
                sector = 5;
            else
                sector = 4;
            end
        else
            quadrant=4;
            if(b < 0)
                sector = 5;
            else
                sector = 6;
            end
        end
        
    else
        if (u_alpha <0)
            quadrant=2;
            if(b < 0)
                sector = 2;
            else
                sector = 3;
            end
        else
            quadrant=1;
            if(b < 0)
                sector = 2;
            else
                sector = 1;
            end
        end
    end
    
    sector = sector;
    
    %%Modulationsfunktionen für Phasen U,V,W
    %%Erzeugung der Aussteuergrade für die Halbbrücken
    %%--> Erzeugung einer "regulary Sampled SVM" erfolgt anschließend durch Abtastung
    %%mit Dreieckszählern in Hardware.
    
    if (sector == 1)
        
        %Quang S.24 and normed to 2/3 U_DC
        u1 = b/(U_max);
        u2 = c/(U_max);
        
        %Quang S.34
        a_U_on = 0.5 + u1*0.5 + u2*0.5;
        a_V_on = 0.5 - u1*0.5 + u2*0.5;
        a_W_on = 0.5 - u1*0.5 - u2*0.5;
    end
    
    
    if ((sector == 2) && (quadrant == 1))
        
        u1 = a/(U_max);
        u2 = (-abs(u_alpha) + 0.5774*abs(u_beta))/(U_max);
        
        a_U_on = 0.5 + u1*0.5 - u2*0.5;
        a_V_on = 0.5 + u1*0.5 + u2*0.5;
        a_W_on = 0.5 - u1*0.5 - u2*0.5;
    end
    
    
    if ((sector == 2) && (quadrant == 2))
        
        u1 = (-abs(u_alpha) + 0.5774*abs(u_beta))/(U_max);
        u2 = a/(U_max);
        
        a_U_on = 0.5 + u1*0.5 - u2*0.5;
        a_V_on = 0.5 + u1*0.5 + u2*0.5;
        a_W_on = 0.5 - u1*0.5 - u2*0.5;
    end
    
    
    if (sector == 3)
        
        u1 = c/(U_max);
        u2 = b/(U_max);
        
        a_U_on=  0.5 - u1*0.5 - u2*0.5;
        a_V_on = 0.5 + u1*0.5 + u2*0.5;
        a_W_on = 0.5 - u1*0.5 + u2*0.5;
    end
    
    if (sector == 4)
        
        u1 = b/(U_max);
        u2 = c/(U_max);
        
        a_U_on = 0.5 - u1*0.5 - u2*0.5;
        a_V_on = 0.5 + u1*0.5 - u2*0.5;
        a_W_on = 0.5 + u1*0.5 + u2*0.5;
    end
    
    
    if ((sector == 5) && (quadrant == 3))
        
        u1 = a/(U_max);
        u2 = (-abs(u_alpha) + 0.5774*abs(u_beta))/(U_max);
        
        a_U_on = 0.5 - u1*0.5 + u2*0.5;
        a_V_on = 0.5 - u1*0.5 - u2*0.5;
        a_W_on = 0.5 + u1*0.5 + u2*0.5;
    end
    
    
    if ((sector == 5) && (quadrant == 4))
        
        u1 =(-abs(u_alpha) + 0.5774*abs(u_beta))/(U_max);
        u2 =  a/(U_max);
        
        a_U_on = 0.5 - u1*0.5 + u2*0.5;
        a_V_on = 0.5 - u1*0.5 - u2*0.5;
        a_W_on = 0.5 + u1*0.5 + u2*0.5;
    end
    
    
    if (sector == 6)
        
        u1 = c/(U_max);
        u2 = b/(U_max);
        
        a_U_on = 0.5 + u1*0.5 + u2*0.5;
        a_V_on = 0.5 - u1*0.5 - u2*0.5;
        a_W_on = 0.5 + u1*0.5 - u2*0.5;
    end
    
    if a_U_on > 1.0
        a_U_on = 1.0;
    end
    if a_V_on > 1.0
        a_V_on = 1.0;
    end
    if a_W_on > 1.0
        a_W_on = 1.0;
    end     
        
    u_a = a_U_on;
    u_b = a_V_on;
    u_c = a_W_on;
